simulink model "compare_plant"  (R2022b)
settings: Solver=VariableStepAuto  StartTime=0.0  StopTime=50  RelTol=1e-3
values from neighbouring files (symbols this model uses):
  alpha_trim = (((Cz_trim + Cz_alp*alpha_0)*(-1*Cm_delm)/Cz_delm) - Cm_0 + (alpha_0*Cm_alpha))/(Cm_alpha + (Cz_alp*(-1*Cm_delm)/Cz_delm))    [variableLoader.m]
  delt_trim = sqrt((T_trim/(ro*Sprop*Cprop/(2*m))) + velocity*velocity)/kMotor    [variableLoader.m]
  delta_m_trim = ((alpha_trim - alpha_0)*Cm_alpha + Cm_0)/(-1*Cm_delm)    [variableLoader.m]
  velocity = 25    [variableLoader.m]
undefined symbols (not defined in the file or in its folder): sigbuilder_block
libraries: cstblocks x10, dspsrcs4 x1

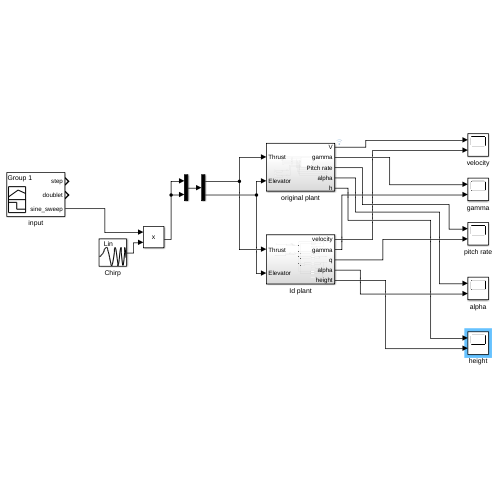
[thumbnail: Simulink's stored preview of the top-level diagram]
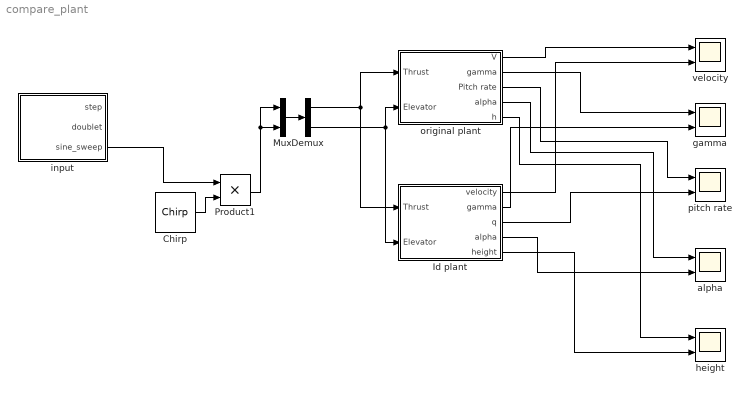
== system compare_plant ==
  Chirp : dspsrcs4/Chirp  sweep=Linear  mode=Unidirectional  f0=0  f1=3  t1=20  Tsweep=20  phase=0  Ts=0.02  spf=1  datatype=Double  OutputFrames=off
  Demux : Demux  Outputs=2
  Id plant : Subsystem
  Mux : Mux  Inputs=2
  Product1 : Product
  alpha : Scope  NumInputPorts=2
  gamma : Scope  NumInputPorts=2
  height : Scope  NumInputPorts=2
  input : Subsystem  Tag=STV Subsys  LoadFcn=sigbuilder_block('load');  StartFcn=sigbuilder_block('start');  StopFcn=sigbuilder_block('stop');  ClipboardFcn=sigbuilder_block('clipboard');  mask(Sigbuilder block){tuvar=[0:10]}
      mask help: Simulink:masks:SigbuilderBlock_MD
      mask init:
      | if ~strcmp(get_param(bdroot(gcbh),'SimulationStatus'),'stopped') tuvar = sigbuilder_block('maskInit'); end
  original plant : Subsystem
  pitch rate : Scope  NumInputPorts=2
  velocity : Scope  NumInputPorts=2
  wires:
  Chirp/1 -> Product1/2
  input/3(sine_sweep) -> Product1/1
  Mux/1 -> Demux/1
  Demux/1 -> Id plant/1(Thrust), original plant/1(Thrust)
  Demux/2 -> original plant/2("Elevator "), Id plant/2("Elevator ")
  original plant/2(gamma) -> gamma/1
  original plant/3(Pitch rate) -> pitch rate/1
  Id plant/3(q) -> pitch rate/2
  original plant/4(alpha) -> alpha/1
  original plant/5(h) -> height/1
  original plant/1(V) -> velocity/1
  Id plant/1(velocity) -> velocity/2
  Id plant/4(alpha) -> alpha/2
  Id plant/2(gamma) -> gamma/2
  Id plant/5(height) -> height/2
  Product1/1 -> Mux/2, Mux/1

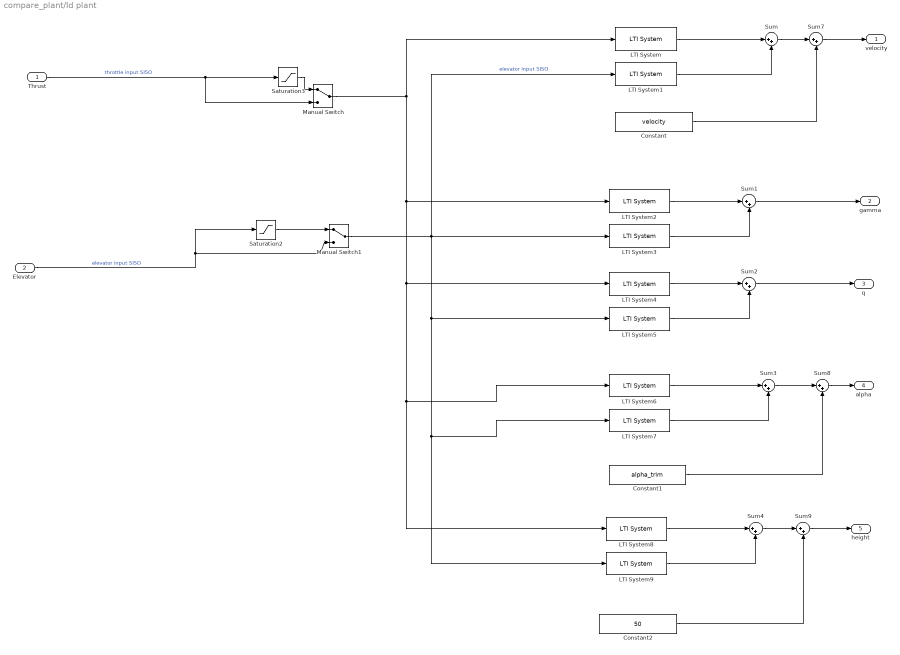
== system compare_plant/Id plant ==
  Thrust : Inport
  "Elevator " : Inport  Port=2
  Constant : Constant  Value=velocity
  Constant1 : Constant  Value=alpha_trim
  Constant2 : Constant  Value=50
  LTI System : cstblocks/LTI System  sys=sys_t_v  IC=[]
  LTI System1 : cstblocks/LTI System  sys=sys_el_v  IC=[]
  LTI System2 : cstblocks/LTI System  sys=sys_t_g  IC=[]
  LTI System3 : cstblocks/LTI System  sys=sys_el_g  IC=[]
  LTI System4 : cstblocks/LTI System  sys=sys_t_pr  IC=[]
  LTI System5 : cstblocks/LTI System  sys=sys_el_pr  IC=[]
  LTI System6 : cstblocks/LTI System  sys=sys_t_a  IC=[]
  LTI System7 : cstblocks/LTI System  sys=sys_el_a  IC=[]
  LTI System8 : cstblocks/LTI System  sys=sys_t_h  IC=[]
  LTI System9 : cstblocks/LTI System  sys=sys_el_h  IC=[]
  Manual Switch : ManualSwitch
  Manual Switch1 : ManualSwitch
  Saturation2 : Saturate  UpperLimit=deg2rad(30)  LowerLimit=-deg2rad(30)
  Saturation3 : Saturate  UpperLimit=1  LowerLimit=0
  Sum{,1..4,7..9} (8 alike) : Sum  Inputs=|++
  velocity : Outport
  gamma : Outport  Port=2
  q : Outport  Port=3
  alpha : Outport  Port=4
  height : Outport  Port=5
  wires:
  Sum1/1 -> gamma/1
  LTI System/1 -> Sum/1
  Sum2/1 -> q/1
  Manual Switch/1 -> LTI System8/1, LTI System6/1, LTI System4/1, LTI System2/1, LTI System/1
  LTI System2/1 -> Sum1/1
  LTI System8/1 -> Sum4/1
  LTI System5/1 -> Sum2/2
  LTI System7/1 -> Sum3/2
  LTI System1/1 -> Sum/2
  LTI System3/1 -> Sum1/2
  LTI System4/1 -> Sum2/1
  LTI System6/1 -> Sum3/1
  LTI System9/1 -> Sum4/2
  Manual Switch1/1 -> LTI System9/1, LTI System7/1, LTI System5/1, LTI System3/1, LTI System1/1  "elevator input SISO"
  Saturation3/1 -> Manual Switch/1
  Saturation2/1 -> Manual Switch1/1
  Thrust/1 -> Manual Switch/2, Saturation3/1  "throttle input SISO"
  "Elevator "/1 -> Saturation2/1, Manual Switch1/2  "elevator input SISO"
  Sum/1 -> Sum7/1
  Sum7/1 -> velocity/1
  Constant/1 -> Sum7/2
  Constant1/1 -> Sum8/2
  Sum3/1 -> Sum8/1
  Sum8/1 -> alpha/1
  Constant2/1 -> Sum9/2
  Sum4/1 -> Sum9/1
  Sum9/1 -> height/1

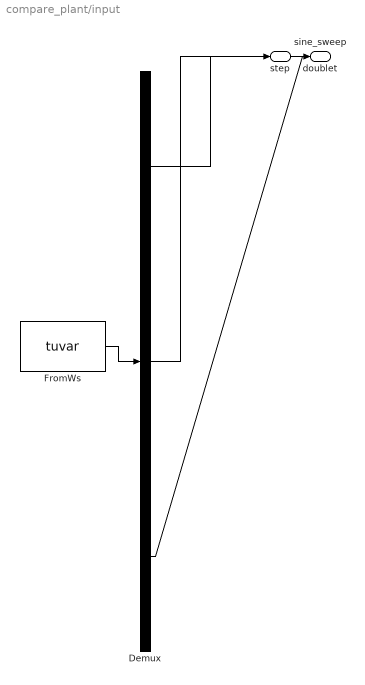
== system compare_plant/input ==
  Demux : Demux  Tag=STV Demux  Outputs=3
  FromWs : FromWorkspace  Tag=STV FromWs  VariableName=tuvar  SampleTime=1/50
      SigBuilderData=|
      | common.afterFinalStr = 'Extrapolate'
      | common.sampleTime = '1/50'
      | dataSet.timeRange = [0 20]
      | dataSet.name = 'Group 1'
      | sbobj.Groups.Name = 'Group 1'
      | sbobj.Groups.Signals(1).Name = 'step'
      | sbobj.Groups.Signals(1).XData = [0 1.98 1.98 5.02 20]
      | sbobj.Groups.Signals(1).YData = [0 0 0.1 0.1 0.1]
      | sbobj.Groups.Signals(2).Name = 'doublet'
      | sbobj.Groups.Signals(2).XData = [0 2 2 2.52 2.52 2.98 2.98 20]
      | sbobj.Groups.Signals(2).YData = [0 0 0.1 0.1 -0.1 -0.1 0 0]
      | sbobj.Groups.Signals(3).Name = 'sine_sweep'
      | sbobj.Groups.Signals(3).XData = [0 1.98 1.98 20]
      | sbobj.Groups.Signals(3).YData = [0 0 0.1 0.1]
      | sbobj.Groups.TimeRange = [0 20]
  step : Outport  Tag=STV Outport
  doublet : Outport  Tag=STV Outport  Port=2
  sine_sweep : Outport  Tag=STV Outport  Port=3
  wires:
  Demux/1 -> step/1
  FromWs/1 -> Demux/1
  Demux/2 -> doublet/1
  Demux/3 -> sine_sweep/1

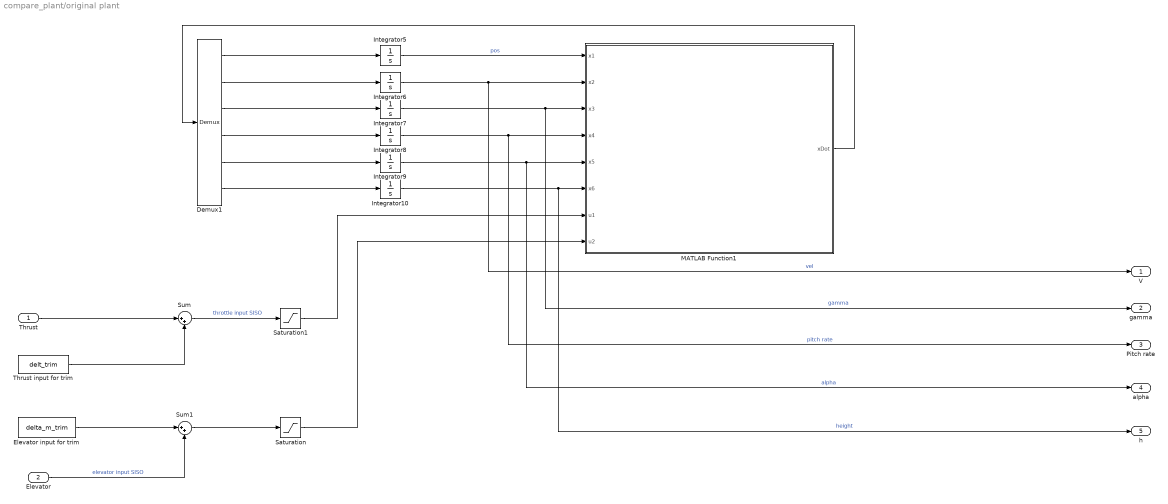
== system compare_plant/original plant ==
  Thrust : Inport
  "Elevator " : Inport  Port=2
  Demux1 : Demux  Outputs=6
  Elevator input for trim : Constant  Value=delta_m_trim
  Integrator10 : Integrator  InitialCondition=50
  Integrator5 : Integrator
  Integrator6 : Integrator  InitialCondition=velocity
  Integrator7 : Integrator
  Integrator8 : Integrator
  Integrator9 : Integrator  InitialCondition=alpha_trim
  MATLAB Function1 : MATLAB Function  TreatAsAtomicUnit=on
  Saturation : Saturate  UpperLimit=deg2rad(30)  LowerLimit=-deg2rad(30)
  Saturation1 : Saturate  UpperLimit=1  LowerLimit=0
  Sum : Sum  Inputs=|++
  Sum1 : Sum  Inputs=|++
  Thrust input for trim : Constant  Value=delt_trim
  V : Outport
  gamma : Outport  Port=2
  Pitch rate : Outport  Port=3
  alpha : Outport  Port=4
  h : Outport  Port=5
  wires:
  Integrator9/1 -> alpha/1, MATLAB Function1/5(x5)  "alpha"
  Sum1/1 -> Saturation/1
  Demux1/2 -> Integrator6/1
  "Elevator "/1 -> Sum1/2  "elevator input SISO"
  Integrator5/1 -> MATLAB Function1/1(x1)  "pos"
  Demux1/3 -> Integrator7/1
  Elevator input for trim/1 -> Sum1/1
  Saturation/1 -> MATLAB Function1/8(u2)
  Thrust/1 -> Sum/1
  Integrator10/1 -> h/1, MATLAB Function1/6(x6)  "height"
  Demux1/5 -> Integrator9/1
  Thrust input for trim/1 -> Sum/2
  Sum/1 -> Saturation1/1  "throttle input SISO"
  Integrator6/1 -> MATLAB Function1/2(x2), V/1  "vel"
  Demux1/1 -> Integrator5/1
  Saturation1/1 -> MATLAB Function1/7(u1)
  Integrator8/1 -> MATLAB Function1/4(x4), Pitch rate/1  "pitch rate"
  Integrator7/1 -> gamma/1, MATLAB Function1/3(x3)  "gamma"
  Demux1/6 -> Integrator10/1
  Demux1/4 -> Integrator8/1
  MATLAB Function1/1(xDot) -> Demux1/1

== matlab function compare_plant/original plant/MATLAB Function1 ==
function xDot = acDynamics_wind(x1,x2,x3,x4,x5,x6,u1,u2)
    
    Cz_alp = 3.45;
    alpha_0 = 0.4712;
    Cz_delm = -0.36;
    Cx_0 = 0.03;
    %ki = 0.055;
    Cm_0 = -0.02338;
    Cm_alpha = -0.38;
    Cm_q = -3.6;
    L = 0.18994;
    Cm_delm = -0.5;
    S = 0.55;
    B = 1.135;
    m = 13.5;
    Sprop = 0.2027;
    ro = 1.2682;
    kMotor = 80;
    Cprop = 1;
    g = 9.8;
    % A/c DYNAMICS
    p = x1;
    V = x2;
    gamma = x3;
    q = x4;
    alpha = x5;
    h = x6;
    dt = u1;
    delm = u2;
    ki = 0.18994/(pi*2.8956*0.1592);
    T = (ro*Sprop*Cprop/(2*m))*((kMotor*dt)^2 - V*V);
    velocity = 25;
    Cz_trim= m*g*cos(0)/(0.5*ro*velocity*velocity*S);
    alpha_trim = (((Cz_trim + Cz_alp*alpha_0)*(-1*Cm_delm)/Cz_delm) - Cm_0 + (alpha_0*Cm_alpha))/(Cm_alpha + (Cz_alp*(-1*Cm_delm)/Cz_delm));
    delta_m_trim = ((alpha_trim - alpha_0)*Cm_alpha + Cm_0)/(-1*Cm_delm);
    Cz_trim = Cz_alp*(alpha_trim - alpha_0) + Cz_delm*delta_m_trim;
    Cx_trim = Cx_0 + ki*Cz_trim^2;
    T_trim =  0.5*ro*velocity*velocity*S*(Cx_trim);

    Cz = Cz_alp*(alpha - alpha_0) + Cz_delm*delm;
    Cx = Cx_0 + ki*Cz^2;
    Cm_G = Cm_0 + Cm_alpha*(alpha - alpha_0) + Cm_q*q*L/V + Cm_delm*delm;
    p_dot = V*cos(gamma); 
    V_dot = (-m*g*sin(gamma) - 0.5*ro*V*V*S*(Cx) + T)/m;
    %V_dot = 0;
    gamma_dot = (m*g*cos(gamma) - 0.5*ro*V*V*S*Cz)/(-m*V);
    
    q_dot = 0.5*ro*V*V*S*L*Cm_G/B;
    
    alpha_dot = q - gamma_dot;
    
    h_dot = V*sin(gamma);
    xDot = [p_dot V_dot gamma_dot q_dot alpha_dot h_dot];
end
